simulink model "Battery_Electrothermal_Model"  (Simulink 7.3)
settings: Solver=ode45  StartTime=0.0  StopTime=10.0  RelTol=1e-3
undefined symbols (not defined in the file or in its folder): C12_SOC_c, C12_SOC_d, C22_SOC_c, C22_SOC_d, C_bat, Cc, Cs, dUdt, R12_SOC_c, R12_SOC_d, R22_SOC_c, R22_SOC_d, Rc, Rs2_SOC_c, Rs2_SOC_d, Ru, SOC_0, SOC_ent, Tc_0, Tf, Ts_0, V_avgC20
libraries: simulink x1
settings Model: Creator=xinfan  LastModifiedBy=xinfan

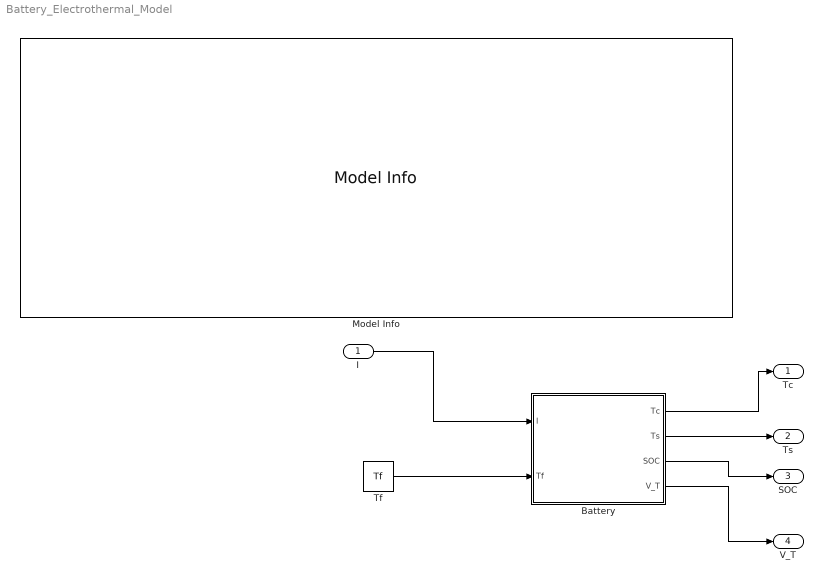
== system Battery_Electrothermal_Model ==
  I : Inport  Interpolate=off
  Battery : Subsystem
  Model Info : simulink/Model-Wide Utilities/Model Info  SystemSampleTime=-1  InitialBlockCM=None  BlockCM=None  Frame=on  DisplayStringWithTags=|  HorizontalTextAlignment=Left  LeftAlignmentValue=0.02  SourceBlockDiagram=Battery_Electrothermal_Model  TagMaxNumber=20
      | COPYRIGHT  2013
      | THE REGENTS OF THE UNIVERSITY OF MICHIGAN
      | ALL RIGHTS RESERVED
      | 
      | PERMISSION IS GRANTED TO USE, COPY AND REDISTRIBUTE THIS SOFTWARE FOR NONCOMMERCIAL EDUCATION AND RESEARCH
      | PURPOSES, SO LONG AS NO FEE IS CHARGED, AND SO LONG AS THE COPYRIGHT NOTICE ABOVE, THIS GRANT OF PERMISSION, 
      | AND THE DISCLAIMER BELOW APPEAR IN ALL COPIES MADE; AND SO LONG AS THE NAME OF THE UNIVERSITY OF MICHIGAN IS NOT 
      | USED IN ANY ADVERTISING OR PUBLICITY PERTAINING TO THE USE OR DISTRIBUTION OF THIS SOFTWARE WITHOUT SPECIFIC, 
      | WRITTEN PRIOR AUTHORIZATION.  PERMISSION TO MODIFY OR OTHERWISE CREATE DERIVATIVE WORKS OF THIS SOFTWARE 
      | IS NOT GRANTED.
      | 
      | THIS USE OF THIS SOFTWARE REQUIRES MATLAB(TM) AND SIMULINK(TM), A LICENSED PRODUCT OF THE MATHWORKS, INC. 
      | THE SOFTWARE USER IS SOLELY RESOPNSIBLE FOR OBTAINTING AN APPROPRIATE LICENSE FOR MATLAB(TM) AND SIMULINK(TM).  
      | NO LICENSE TO MATLAB(TM) AND SIMULINK(TM) IS GRANTED, INFERRED OR IMPLIED BY THE DISTRIBUTION OF THIS SOFTWARE.
      | 
      | THIS SOFTWARE IS PROVIDED AS IS, WITHOUT REPRESENTATION AS TO ITS FITNESS FOR ANY PURPOSE, AND WITHOUT WARRANTY 
      | OF ANY KIND, EITHER EXPRESS OR IMPLIED, INCLUDING WITHOUT LIMITATION THE IMPLIED WARRANTIES OF MERCHANTABILITY AND
      | FITNESS FOR A PARTICULAR PURPOSE. THE REGENTS OF THE UNIVERSITY OF MICHIGAN SHALL NOT BE LIABLE FOR ANY DAMAGES,
      | INCLUDING SPECIAL, INDIRECT, INCIDENTAL, OR CONSEQUENTIAL DAMAGES, WITH RESPECT TO ANY CLAIM ARISING OUT OF OR IN
      | CONNECTION WITH THE USE OF THE SOFTWARE, EVEN IF IT HAS BEEN OR IS HEREAFTER ADVISED OF THE POSSIBILITY OF SUCH 
      | DAMAGES.
  Tf : Constant  Value=Tf  OutDataType=fixdt(1, 16)  OutScaling=2^0
  Tc : Outport  OutDataType=fixdt(1, 16)  OutScaling=2^0
  Ts : Outport  Port=2  OutDataType=fixdt(1, 16)  OutScaling=2^0
  SOC : Outport  Port=3  OutDataType=fixdt(1, 16)  OutScaling=2^0
  V_T : Outport  Port=4  OutDataType=fixdt(1, 16)  OutScaling=2^0
  wires:
  Tf/1 -> Battery/2(Tf)
  I/1 -> Battery/1(I)
  Battery/1(Tc) -> Tc/1
  Battery/2(Ts) -> Ts/1
  Battery/3(SOC) -> SOC/1
  Battery/4(V_T) -> V_T/1

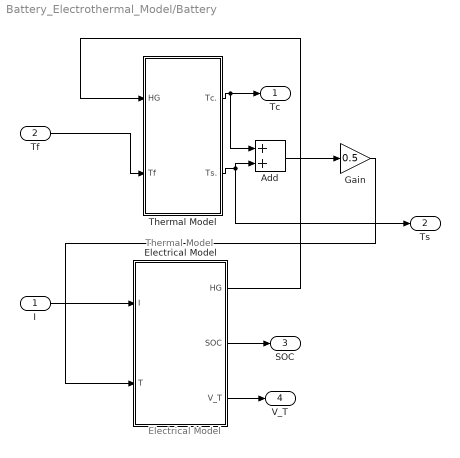
== system Battery_Electrothermal_Model/Battery ==
  note: Electrical Model
  note: Thermal Model
  I : Inport  Interpolate=off
  Tf : Inport  Port=2
  Add : Sum  OutDataType=fixdt(1, 16)  OutScaling=2^-10
  Electrical Model : Subsystem  Tag=electrical
  Gain : Gain  Gain=0.5  ParameterDataType=fixdt(1, 16)  ParameterScaling=2^0  OutDataType=fixdt(1, 16)  OutScaling=2^0
  Thermal Model : Subsystem
  Tc : Outport
  Ts : Outport  Port=2
  SOC : Outport  Port=3
  V_T : Outport  Port=4
  wires:
  Electrical Model/3(V_T) -> V_T/1
  I/1 -> Electrical Model/1(I)
  Thermal Model/1(Tc.) -> Add/1, Tc/1
  Electrical Model/2(SOC) -> SOC/1
  Electrical Model/1(HG) -> Thermal Model/1(HG)
  Thermal Model/2(Ts.) -> Add/2, Ts/1
  Add/1 -> Gain/1
  Tf/1 -> Thermal Model/2(Tf)
  Gain/1 -> Electrical Model/2(T)

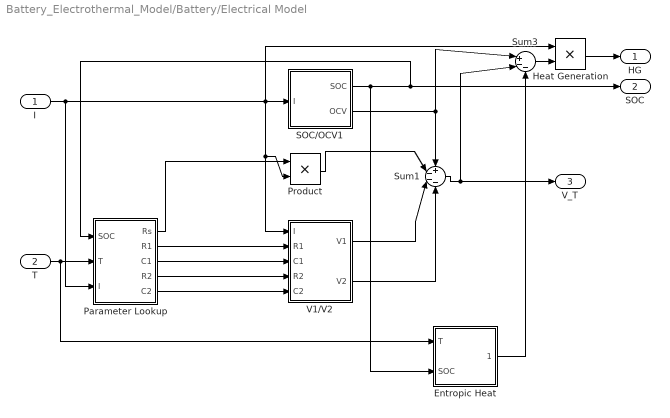
== system Battery_Electrothermal_Model/Battery/Electrical Model ==
  I : Inport
  T : Inport  Port=2
  Entropic Heat : Subsystem
  Heat Generation : Product  RndMeth=Zero
  Parameter Lookup : Subsystem
  Product : Product  RndMeth=Zero
  SOC/OCV1 : Subsystem
  Sum1 : Sum  Inputs=+---
  Sum3 : Sum  Inputs=|+--
  V1/V2 : Subsystem
  HG : Outport
  SOC : Outport  Port=2
  V_T : Outport  Port=3
  wires:
  I/1 -> Parameter Lookup/3(I), Heat Generation/1, Product/2, V1/V2/1(I), SOC/OCV1/1(I)
  V1/V2/1(V1) -> Sum1/3
  Sum1/1 -> V_T/1, Sum3/2
  SOC/OCV1/1(SOC) -> Parameter Lookup/1(SOC), SOC/1, Entropic Heat/2(SOC)
  Product/1 -> Sum1/2
  Sum3/1 -> Heat Generation/2
  SOC/OCV1/2(OCV) -> Sum3/1, Sum1/1
  Parameter Lookup/1(Rs) -> Product/1
  Parameter Lookup/2(R1) -> V1/V2/2(R1)
  Parameter Lookup/4(R2) -> V1/V2/4(R2)
  T/1 -> Parameter Lookup/2(T), Entropic Heat/1(T)
  Heat Generation/1 -> HG/1
  Parameter Lookup/3(C1) -> V1/V2/3(C1)
  Parameter Lookup/5(C2) -> V1/V2/5(C2)
  V1/V2/2(V2) -> Sum1/4
  Entropic Heat/1(HG_ent) -> Sum3/3

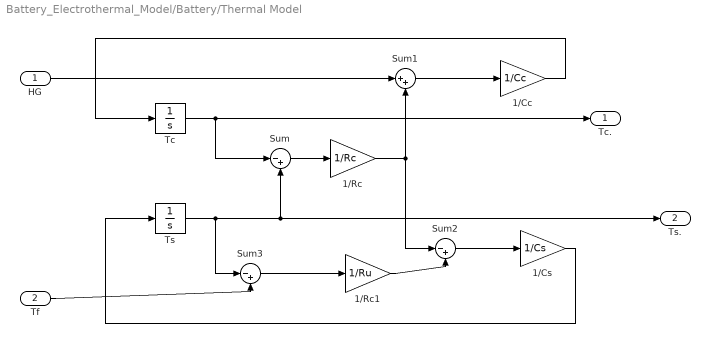
== system Battery_Electrothermal_Model/Battery/Thermal Model ==
  HG : Inport
  Tf : Inport  Port=2
  1/Cc : Gain  Gain=1/Cc
  1/Cs : Gain  Gain=1/Cs
  1/Rc : Gain  Gain=1/Rc
  1/Rc1 : Gain  Gain=1/Ru
  Sum : Sum  Inputs=|-+
  Sum1 : Sum  Inputs=|++
  Sum2 : Sum  Inputs=|-+
  Sum3 : Sum  Inputs=|-+
  Tc : Integrator  InitialCondition=Tc_0
  Ts : Integrator  InitialCondition=Ts_0
  Tc. : Outport
  Ts. : Outport  Port=2
  wires:
  HG/1 -> Sum1/1
  Tf/1 -> Sum3/2
  Ts/1 -> Sum3/1, Sum/2, Ts./1
  Tc/1 -> Sum/1, Tc./1
  Sum/1 -> 1/Rc/1
  1/Rc/1 -> Sum2/1, Sum1/2
  Sum1/1 -> 1/Cc/1
  1/Cc/1 -> Tc/1
  Sum2/1 -> 1/Cs/1
  1/Cs/1 -> Ts/1
  Sum3/1 -> 1/Rc1/1
  1/Rc1/1 -> Sum2/2

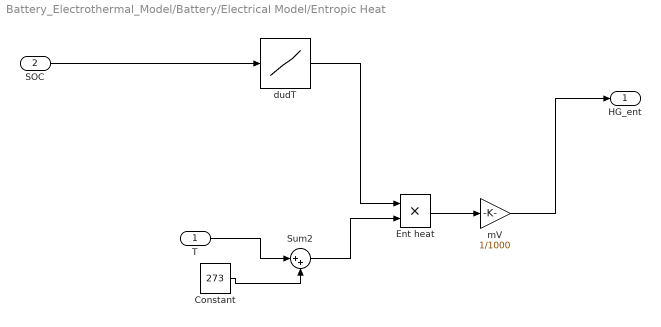
== system Battery_Electrothermal_Model/Battery/Electrical Model/Entropic Heat ==
  T : Inport  OutDataType=fixdt(1, 16)  OutScaling=2^0
  SOC : Inport  Port=2  OutDataType=fixdt(1, 16)  OutScaling=2^0
  Constant : Constant  Value=273  OutDataType=fixdt(1, 16)  OutScaling=2^0
  Ent heat : Product  OutDataType=fixdt(1, 16)  OutScaling=2^0  RndMeth=Zero
  Sum2 : Sum  Inputs=|++  OutDataType=fixdt(1, 16)  OutScaling=2^0
  dudT : Lookup  InputValues=SOC_ent  Table=dUdt  OutDataType=fixdt(1, 16)  OutScaling=2^0
  mV : Gain  Gain=1/1000  ParameterDataType=fixdt(1, 16)  ParameterScaling=2^0  OutDataType=fixdt(1, 16)  OutScaling=2^0
  HG_ent : Outport  OutDataType=fixdt(1, 16)  OutScaling=2^0
  wires:
  Sum2/1 -> Ent heat/2
  Constant/1 -> Sum2/2
  T/1 -> Sum2/1
  dudT/1 -> Ent heat/1
  Ent heat/1 -> mV/1
  SOC/1 -> dudT/1
  mV/1 -> HG_ent/1

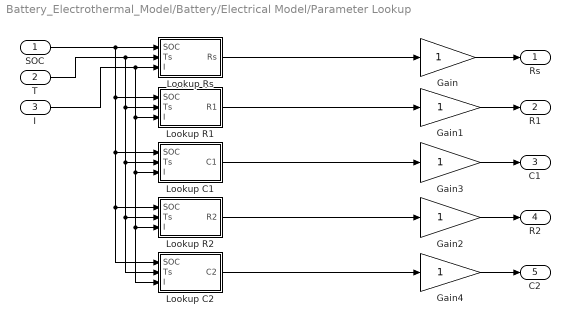
== system Battery_Electrothermal_Model/Battery/Electrical Model/Parameter Lookup ==
  SOC : Inport
  T : Inport  Port=2
  I : Inport  Port=3
  Gain{,1..4} (5 alike) : Gain
  Lookup C1 : Subsystem
  Lookup C2 : Subsystem
  Lookup R1 : Subsystem
  Lookup R2 : Subsystem
  Lookup Rs : Subsystem
  Rs : Outport
  R1 : Outport  Port=2
  C1 : Outport  Port=3
  R2 : Outport  Port=4
  C2 : Outport  Port=5
  wires:
  SOC/1 -> Lookup Rs/1(SOC), Lookup R1/1(SOC), Lookup C1/1(SOC), Lookup R2/1(SOC), Lookup C2/1(SOC)
  T/1 -> Lookup Rs/2(Ts), Lookup R1/2(Ts), Lookup C1/2(Ts), Lookup R2/2(Ts), Lookup C2/2(Ts)
  I/1 -> Lookup Rs/3(I), Lookup R1/3(I), Lookup C1/3(I), Lookup R2/3(I), Lookup C2/3(I)
  Lookup Rs/1(Rs) -> Gain/1
  Gain3/1 -> C1/1
  Lookup C2/1(C2) -> Gain4/1
  Gain4/1 -> C2/1
  Gain2/1 -> R2/1
  Lookup R2/1(R2) -> Gain2/1
  Gain1/1 -> R1/1
  Gain/1 -> Rs/1
  Lookup R1/1(R1) -> Gain1/1
  Lookup C1/1(C1) -> Gain3/1

== system Battery_Electrothermal_Model/Battery/Electrical Model/SOC/OCV1 ==
  I : Inport
  Avg : Lookup  InputValues=[0:0.001:1]  Table=V_avgC20  LookUpMeth=Interpolation-Use End Values
  Gain1 : Gain  Gain=-1/(3600*C_bat)
  Integrator : Integrator  InitialCondition=SOC_0
  SOC : Outport
  OCV : Outport  Port=2
  wires:
  Integrator/1 -> SOC/1, Avg/1
  Avg/1 -> OCV/1
  I/1 -> Gain1/1
  Gain1/1 -> Integrator/1

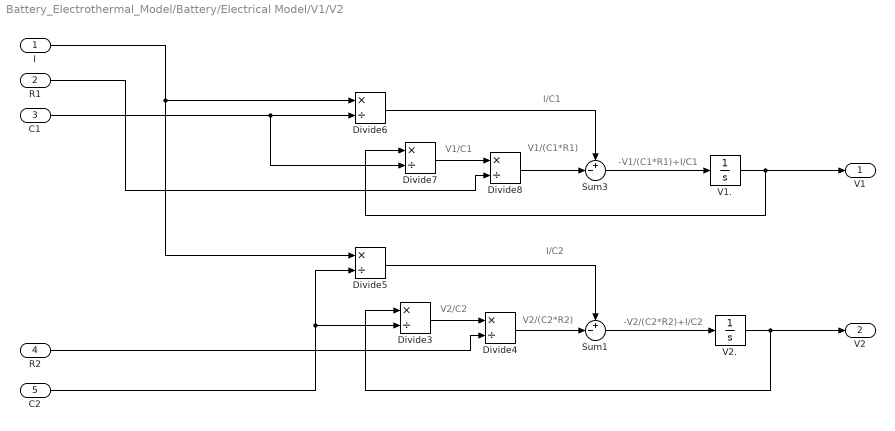
== system Battery_Electrothermal_Model/Battery/Electrical Model/V1/V2 ==
  note: V2/(C2*R2)
  note: -V2/(C2*R2)+I/C2
  note: V2/C2
  note: I/C2
  note: V1/(C1*R1)
  note: I/C1
  note: -V1/(C1*R1)+I/C1
  note: V1/C1
  I : Inport
  R1 : Inport  Port=2
  C1 : Inport  Port=3
  R2 : Inport  Port=4
  C2 : Inport  Port=5
  Divide{3..8} (6 alike) : Product  Inputs=*/  RndMeth=Zero
  Sum1 : Sum  Inputs=+-|
  Sum3 : Sum  Inputs=+-|
  V1. : Integrator
  V2. : Integrator
  V1 : Outport
  V2 : Outport  Port=2
  wires:
  C1/1 -> Divide6/2, Divide7/2
  V2./1 -> Divide3/1, V2/1
  Divide4/1 -> Sum1/2
  Sum1/1 -> V2./1
  C2/1 -> Divide5/2, Divide3/2
  Divide3/1 -> Divide4/1
  R2/1 -> Divide4/2
  Divide5/1 -> Sum1/1
  V1./1 -> Divide7/1, V1/1
  Divide8/1 -> Sum3/2
  Sum3/1 -> V1./1
  Divide6/1 -> Sum3/1
  Divide7/1 -> Divide8/1
  I/1 -> Divide5/1, Divide6/1
  R1/1 -> Divide8/2

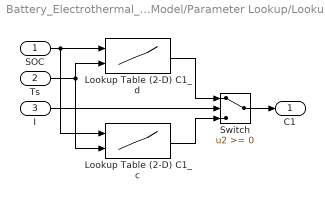
== system Battery_Electrothermal_Model/Battery/Electrical Model/Parameter Lookup/Lookup C1 ==
  SOC : Inport
  Ts : Inport  Port=2
  I : Inport  Port=3
  Lookup Table (2-D) C1_c : Lookup2D  RowIndex=SOC_Temp_c  ColumnIndex=Temp  Table=C12_SOC_c
  Lookup Table (2-D) C1_d : Lookup2D  RowIndex=SOC_Temp_d  ColumnIndex=Temp  Table=C12_SOC_d
  Switch : Switch
  C1 : Outport
  wires:
  Ts/1 -> Lookup Table (2-D) C1_c/2, Lookup Table (2-D) C1_d/2
  SOC/1 -> Lookup Table (2-D) C1_c/1, Lookup Table (2-D) C1_d/1
  Lookup Table (2-D) C1_c/1 -> Switch/3
  Lookup Table (2-D) C1_d/1 -> Switch/1
  Switch/1 -> C1/1
  I/1 -> Switch/2

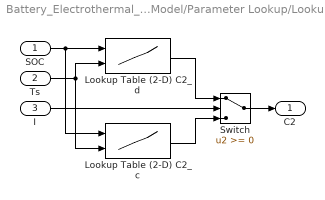
== system Battery_Electrothermal_Model/Battery/Electrical Model/Parameter Lookup/Lookup C2 ==
  SOC : Inport
  Ts : Inport  Port=2
  I : Inport  Port=3
  Lookup Table (2-D) C2_c : Lookup2D  RowIndex=SOC_Temp_c  ColumnIndex=Temp  Table=C22_SOC_c  LookUpMeth=Interpolation-Use End Values
  Lookup Table (2-D) C2_d : Lookup2D  RowIndex=SOC_Temp_d  ColumnIndex=Temp  Table=C22_SOC_d  LookUpMeth=Interpolation-Use End Values
  Switch : Switch
  C2 : Outport
  wires:
  Switch/1 -> C2/1
  Lookup Table (2-D) C2_d/1 -> Switch/1
  Lookup Table (2-D) C2_c/1 -> Switch/3
  SOC/1 -> Lookup Table (2-D) C2_c/1, Lookup Table (2-D) C2_d/1
  Ts/1 -> Lookup Table (2-D) C2_c/2, Lookup Table (2-D) C2_d/2
  I/1 -> Switch/2

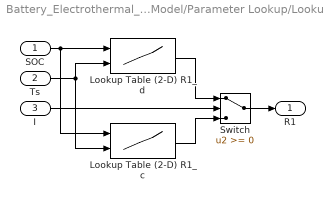
== system Battery_Electrothermal_Model/Battery/Electrical Model/Parameter Lookup/Lookup R1 ==
  SOC : Inport
  Ts : Inport  Port=2
  I : Inport  Port=3
  Lookup Table (2-D) R1_c : Lookup2D  RowIndex=SOC_Temp_c  ColumnIndex=Temp  Table=R12_SOC_c
  Lookup Table (2-D) R1_d : Lookup2D  RowIndex=SOC_Temp_d  ColumnIndex=Temp  Table=R12_SOC_d
  Switch : Switch
  R1 : Outport
  wires:
  Ts/1 -> Lookup Table (2-D) R1_d/2, Lookup Table (2-D) R1_c/2
  SOC/1 -> Lookup Table (2-D) R1_d/1, Lookup Table (2-D) R1_c/1
  Lookup Table (2-D) R1_c/1 -> Switch/3
  Lookup Table (2-D) R1_d/1 -> Switch/1
  I/1 -> Switch/2
  Switch/1 -> R1/1

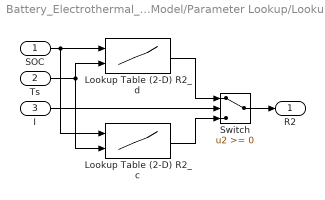
== system Battery_Electrothermal_Model/Battery/Electrical Model/Parameter Lookup/Lookup R2 ==
  SOC : Inport
  Ts : Inport  Port=2
  I : Inport  Port=3
  Lookup Table (2-D) R2_c : Lookup2D  RowIndex=SOC_Temp_c  ColumnIndex=Temp  Table=R22_SOC_c  LookUpMeth=Interpolation-Use End Values
  Lookup Table (2-D) R2_d : Lookup2D  RowIndex=SOC_Temp_d  ColumnIndex=Temp  Table=R22_SOC_d  LookUpMeth=Interpolation-Use End Values
  Switch : Switch
  R2 : Outport
  wires:
  Switch/1 -> R2/1
  I/1 -> Switch/2
  Lookup Table (2-D) R2_d/1 -> Switch/1
  Lookup Table (2-D) R2_c/1 -> Switch/3
  SOC/1 -> Lookup Table (2-D) R2_d/1, Lookup Table (2-D) R2_c/1
  Ts/1 -> Lookup Table (2-D) R2_d/2, Lookup Table (2-D) R2_c/2

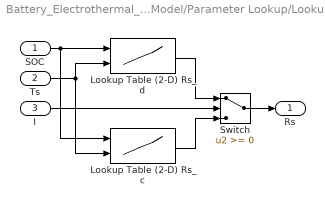
== system Battery_Electrothermal_Model/Battery/Electrical Model/Parameter Lookup/Lookup Rs ==
  SOC : Inport
  Ts : Inport  Port=2
  I : Inport  Port=3
  Lookup Table (2-D) Rs_c : Lookup2D  RowIndex=SOC_Temp_c  ColumnIndex=Temp  Table=Rs2_SOC_c
  Lookup Table (2-D) Rs_d : Lookup2D  RowIndex=SOC_Temp_d  ColumnIndex=Temp  Table=Rs2_SOC_d
  Switch : Switch
  Rs : Outport
  wires:
  Switch/1 -> Rs/1
  I/1 -> Switch/2
  Lookup Table (2-D) Rs_d/1 -> Switch/1
  Lookup Table (2-D) Rs_c/1 -> Switch/3
  SOC/1 -> Lookup Table (2-D) Rs_d/1, Lookup Table (2-D) Rs_c/1
  Ts/1 -> Lookup Table (2-D) Rs_d/2, Lookup Table (2-D) Rs_c/2
